simulink model "Parking"  (R2024a)
settings: Solver=VariableStepAuto  StartTime=0.0  StopTime=10.0  RelTol=1e-3
undefined symbols (not defined in the file): Traffic_Info
libraries: CarMaker4SL x56, slpidlib x1
settings Model: Creator=User  LastModifiedBy=User

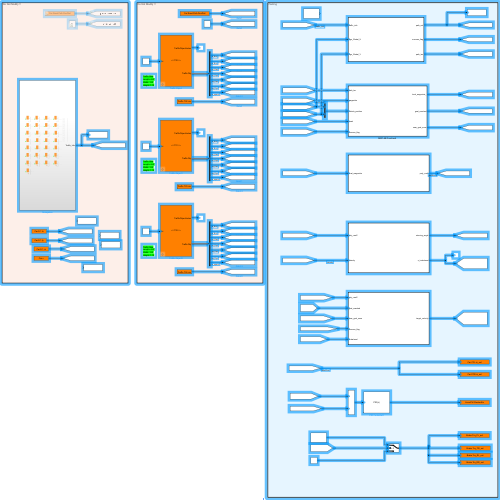
[thumbnail: Simulink's stored preview of the top-level diagram]
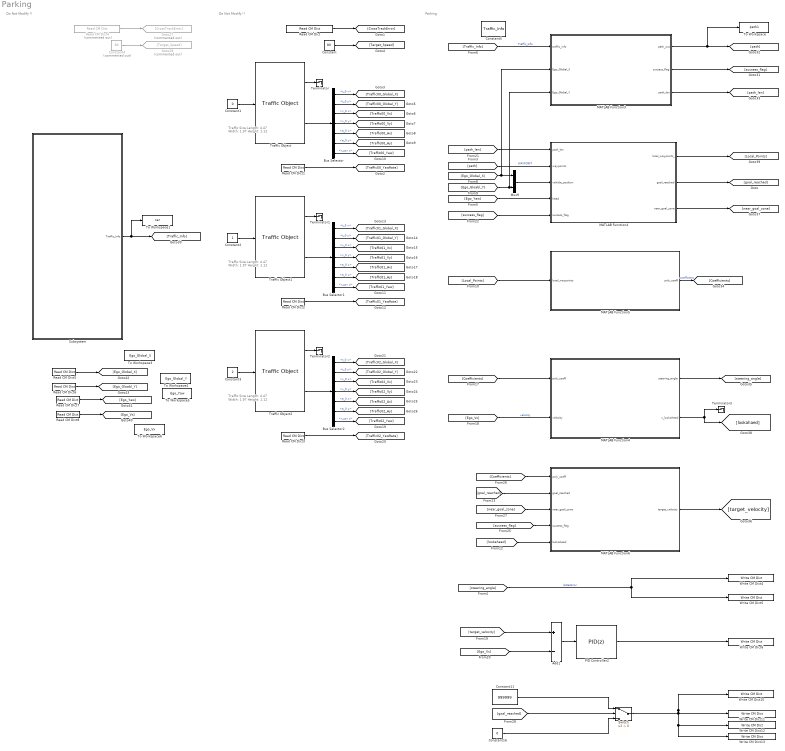
== system Parking ==
  note: Do Not Modify !!
  note: Traffic Size
      | Length: 4.47
      | Width: 1.97
      | Height: 1.12
  note: Traffic Size
      | Length: 4.47
      | Width: 1.97
      | Height: 1.12
  note: Traffic Size
      | Length: 4.47
      | Width: 1.97
      | Height: 1.12
  note: Do Not Modify !!
  note: Parking
  Add1 : Sum  Inputs=+-
  Bus Selector : BusSelector  OutputSignals=t_0 x,t_0 y,v_0 x,v_0 y,a_0 x,a_0 y,r_zyx z
  Bus Selector1 : BusSelector  OutputSignals=t_0 x,t_0 y,v_0 x,v_0 y,a_0 x,a_0 y,r_zyx z
  Bus Selector2 : BusSelector  OutputSignals=t_0 x,t_0 y,v_0 x,v_0 y,a_0 x,a_0 y,r_zyx z
  Constant : Constant  Value=80
  Constant1 : Constant  Value=0
  Constant11 : Constant  Value=999999
  Constant16 : Constant  Value=0
  Constant2 : Constant
  Constant3 : Constant  Value=2
  Constant4 : Constant  Commented=on  Value=80
  Constant5 : Constant  Value=Traffic_Info
  Goto27 : Goto  Commented=on  GotoTag=CrossTrackError
  Goto29 : Goto  Commented=on  GotoTag=Target_Speed
  MATLAB Function3 : MATLAB Function  TreatAsAtomicUnit=on
  MATLAB Function4 : MATLAB Function  TreatAsAtomicUnit=on
  "MATLAB Function4 " : MATLAB Function  TreatAsAtomicUnit=on
  MATLAB Function5 : MATLAB Function  TreatAsAtomicUnit=on
  MATLAB Function6 : MATLAB Function  TreatAsAtomicUnit=on
  Mux9 : Mux  Inputs=2
  PID Controller2 : slpidlib/PID Controller  Controller=PID  Form=Parallel  TimeDomain=Discrete-time  UseExternalTs=off  SampleTime=-1  IntegratorMethod=Forward Euler  FilterMethod=Forward Euler  ControllerParametersSource=internal  P=3  I=0.00  UseKiTs=off  D=0.1  UseExternalDerivativeSource=off  N=100  UseFilter=off  TunerSelectOption=Transfer Function Based (PID Tuner App)  InitialConditionSource=internal  InitialConditionForIntegrator=0  InitialConditionForFilter=0  DifferentiatorICPrevScaledInput=0  ExternalReset=none  TrackingMode=off  Kt=1  LimitOutput=off  SatLimitsSource=internal  UpperSaturationLimit=inf  LowerSaturationLimit=-inf  LinearizeAsGain=on  AntiWindupMode=none  Kb=1  LimitIntegrator=off  UpperIntegratorSaturationLimit=inf  LowerIntegratorSaturationLimit=-inf  POutMin=[]  POutMax=[]  IOutMin=[]  IOutMax=[]  DOutMin=[]  DOutMax=[]  NOutMin=[]  NOutMax=[]  SumOutMin=[]  SumOutMax=[]  SaturationOutMin=[]  SaturationOutMax=[]  PParamMin=[]  PParamMax=[]  IParamMin=[]  IParamMax=[]  DParamMin=[]  DParamMax=[]  NParamMin=[]  NParamMax=[]  KbParamMin=[]  KbParamMax=[]  KtParamMin=[]  KtParamMax=[]  KbOutMin=[]  KbOutMax=[]  KtOutMin=[]  KtOutMax=[]  IntegratorOutMin=[]  IntegratorOutMax=[]  FilterOutMin=[]  FilterOutMax=[]  SumI1OutMin=[]  SumI1OutMax=[]  SumI2OutMin=[]  SumI2OutMax=[]  SumI3OutMin=[]  SumI3OutMax=[]  SumI4OutMin=[]  SumI4OutMax=[]  SumDOutMin=[]  SumDOutMax=[]  DifferentiatorOutMin=[]  DifferentiatorOutMax=[]  FilterDiffOutCoefMin=[]  FilterDiffOutCoefMax=[]  ReciprocalOutMin=[]  ReciprocalOutMax=[]  SumDenOutMin=[]  SumDenOutMax=[]  SumNumOutMin=[]  SumNumOutMax=[]  DivideOutMin=[]  DivideOutMax=[]  UdiffTsProdOutMin=[]  UdiffTsProdOutMax=[]  NTsProdOutMin=[]  NTsProdOutMax=[]  UintegralTsProdOutMin=[]  UintegralTsProdOutMax=[]  UngainTsProdOutMin=[]  UngainTsProdOutMax=[]  ClampingZeroOutDataTypeStr=Inherit: Inherit via back propagation  ClampingZeroOutMin=[]  ClampingZeroOutMax=[]  FilterDenConstantOutDataTypeStr=Inherit: Inherit via back propagation  FilterDenConstantOutMin=[]  FilterDenConstantOutMax=[]  PCopyOutDataTypeStr=Inherit: Inherit via back propagation  PCopyOutMin=[]  PCopyOutMax=[]  NCopyOutDataTypeStr=Inherit: Inherit via back propagation  NCopyOutMin=[]  NCopyOutMax=[]  IntegratorContinuousStateAttributes=''  IntegratorStateMustResolveToSignalObject=off  IntegratorRTWStateStorageClass=Auto  FilterContinuousStateAttributes=''  FilterStateMustResolveToSignalObject=off  FilterRTWStateStorageClass=Auto  ParallelPVariant=InternalParameters  IdealPVariant=Disabled  IVariant=InternalParameters  DVariant=InternalParameters  IntegratorVariant=Discrete  SatVariant=Disabled  AWVariant=Passthrough  PCopyVariant=Disabled  TRVariant=Disabled  FdbkBlocksVariant=Forward  IdealPFdbkVariant=Disabled  SatFdbkVariant=Disabled  DerivativeFilterVariant=Differentiator  NVariant=Passthrough  NCopyVariant=Disabled_SignalSpec  FilterICVariant=InternalICsDifferentiator  IntegratorICVariant=InternalICs  ExternalResetVariant=Disabled  TRSumVariant=Passthrough  SumFdbkVariant=Disabled  SumVariant=Sum_PID  TsampFilterVariant=InternalTs  TsampNgainVariant=Passthrough  TsampIntegralVariant=Disabled_SignalSpec  ExternalSaturationOutDataTypeStr=Inherit: Same as second input  DerivativeSourceVariant=ErrorSignal
  Read CM Dict : CarMaker4SL/Read CM Dict  xname=Car.Road.Path.DevDist  xsync=off  xstime=Inherited
  Read CM Dict1 : CarMaker4SL/Read CM Dict  xname=Traffic.T22.rzv  xsync=off  xstime=Inherited
  Read CM Dict2 : CarMaker4SL/Read CM Dict  xname=Traffic.T23.rzv  xsync=off  xstime=Inherited
  Read CM Dict3 : CarMaker4SL/Read CM Dict  xname=Traffic.T24.rzv  xsync=off  xstime=Inherited
  Read CM Dict4 : CarMaker4SL/Read CM Dict  Commented=on  xname=Car.Road.Path.DevDist  xsync=off  xstime=Inherited
  Read CM Dict5 : CarMaker4SL/Read CM Dict  xname=Car.Fr1.tx  xsync=off  xstime=Inherited
  Read CM Dict6 : CarMaker4SL/Read CM Dict  xname=Car.Fr1.ty  xsync=off  xstime=Inherited
  Read CM Dict7 : CarMaker4SL/Read CM Dict  xname=Car.Fr1.rz  xsync=off  xstime=Inherited
  Read CM Dict8 : CarMaker4SL/Read CM Dict  xname=Car.v  xsync=off  xstime=Inherited
  Subsystem : Subsystem
  Switch : Switch  Criteria=u2 > Threshold  SaturateOnIntegerOverflow=off  InputSameDT=off
  Terminator{,1..3} (4 alike) : Terminator
  To Workspace : ToWorkspace  VariableName=path1  SaveFormat=Structure With Time  SampleTime=-1
  To Workspace1 : ToWorkspace  VariableName=car  SaveFormat=Timeseries  SampleTime=-1
  To Workspace3 : ToWorkspace  VariableName=Ego_Global_X  SaveFormat=Structure With Time  SampleTime=-1
  To Workspace4 : ToWorkspace  VariableName=Ego_Global_Y  SaveFormat=Structure With Time  SampleTime=-1
  To Workspace5 : ToWorkspace  VariableName=Ego_Yaw  SaveFormat=Structure With Time  SampleTime=-1
  To Workspace6 : ToWorkspace  VariableName=Ego_Vx  SaveFormat=Structure With Time  SampleTime=-1
  Traffic Object : CarMaker4SL/Traffic Object  xname=T00  ximode=Traffic Id  xstime=Inherited
      settings: SourceProductName=CarMaker4SL
  Traffic Object1 : CarMaker4SL/Traffic Object  xname=T01  ximode=Traffic Id  xstime=Inherited
      settings: SourceProductName=CarMaker4SL
  Traffic Object2 : CarMaker4SL/Traffic Object  xname=T02  ximode=Traffic Id  xstime=Inherited
      settings: SourceProductName=CarMaker4SL
  Write CM Dict10 : CarMaker4SL/Write CM Dict  xname=Brake.Trq_FL_ext  xsync=off
  Write CM Dict11 : CarMaker4SL/Write CM Dict  xname=Brake.Trq_FR_ext  xsync=off
  Write CM Dict12 : CarMaker4SL/Write CM Dict  xname=Brake.Trq_RL_ext  xsync=off
  Write CM Dict13 : CarMaker4SL/Write CM Dict  xname=Brake.Trq_RR_ext  xsync=off
  Write CM Dict4 : CarMaker4SL/Write CM Dict  xname=Car.CFL.rz_ext  xsync=off
  Write CM Dict5 : CarMaker4SL/Write CM Dict  xname=Car.CFR.rz_ext  xsync=off
  Write CM Dict6 : CarMaker4SL/Write CM Dict  xname=AccelCtrl.DesiredAx  xsync=off
  wires:
  [steering_angle] -> Write CM Dict5/1, Write CM Dict4/1  "latterError"
  [Traffic_Info] -> MATLAB Function3/1(traffic_info)  "Traffic_Info"
  [Ego_Yaw] -> "MATLAB Function4 "/4(head)
  [Coefficients] -> MATLAB Function4/1(poly_coeff)
  Traffic Object2/1 -> Terminator2/1
  Read CM Dict5/1 -> [Ego_Global_X]
  Constant11/1 -> Switch/1
  [success_flag] -> "MATLAB Function4 "/5(success_flag)
  Bus Selector1/1 -> [Traffic01_Global_X]  "<t_0 x>"
  [goal_reached] -> MATLAB Function6/2(goal_reached)
  [success_flag] -> MATLAB Function6/4(success_flag)
  Constant16/1 -> Switch/3
  Read CM Dict8/1 -> [Ego_Vx]
  Read CM Dict3/1 -> [Traffic02_YawRate]
  MATLAB Function3/3(path_len) -> [path_len]
  "MATLAB Function4 "/1(local_waypoints_) -> [Local_Points]
  MATLAB Function5/1(poly_coeff) -> [Coefficients]  "coefficient"
  Bus Selector2/3 -> [Traffic02_Vx]  "<v_0 x>"
  Subsystem/1(Traffic_Info) -> To Workspace1/1, [Traffic_Info]
  [Coefficients] -> MATLAB Function6/1(poly_coeff)
  Bus Selector/6 -> [Traffic00_Ay]  "<a_0 y>"
  Constant4/1 -> Goto29/1
  Bus Selector2/6 -> [Traffic02_Ay]  "<a_0 y>"
  [path_len] -> "MATLAB Function4 "/1(path_len)
  Add1/1 -> PID Controller2/1
  Traffic Object/1 -> Terminator/1
  MATLAB Function3/2(success_flag) -> [success_flag]
  Bus Selector1/5 -> [Traffic01_Ax]  "<a_0 x>"
  [path] -> "MATLAB Function4 "/2(waypoints)  "WAYPOINT"
  Read CM Dict7/1 -> [Ego_Yaw]
  MATLAB Function4/2(x_lookahead) -> Terminator3/1, [lookahaed]
  Bus Selector1/3 -> [Traffic01_Vx]  "<v_0 x>"
  MATLAB Function6/1(target_velocity) -> [target_velocity]
  [target_velocity] -> Add1/1
  Mux9/1 -> "MATLAB Function4 "/3(vehicle_position)
  "MATLAB Function4 "/2(goal_reached) -> [goal_reached]
  [near_goal_zone] -> MATLAB Function6/3(near_goal_zone)
  Constant3/1 -> Traffic Object2/1
  Bus Selector2/2 -> [Traffic02_Global_Y]  "<t_0 y>"
  [Ego_Global_X] -> MATLAB Function3/2(Ego_Global_X), Mux9/1
  "MATLAB Function4 "/3(near_goal_zone) -> [near_goal_zone]
  Read CM Dict6/1 -> [Ego_Gloabl_Y]
  Read CM Dict2/1 -> [Traffic01_YawRate]
  [Ego_Vx] -> Add1/2
  Bus Selector/7 -> [Traffic00_Yaw]  "<r_zyx z>"
  Bus Selector2/5 -> [Traffic02_Ax]  "<a_0 x>"
  [goal_reached] -> Switch/2
  Traffic Object1/2 -> Bus Selector1/1
  Traffic Object1/1 -> Terminator1/1
  Bus Selector/2 -> [Traffic00_Global_Y]  "<t_0 y>"
  [lookahaed] -> MATLAB Function6/5(lookahead)
  Bus Selector/1 -> [Traffic00_Global_X]  "<t_0 x>"
  [Local_Points] -> MATLAB Function5/1(local_waypoints)
  Bus Selector1/4 -> [Traffic01_Vy]  "<v_0 y>"
  MATLAB Function4/1(steering_angle) -> [steering_angle]
  Traffic Object2/2 -> Bus Selector2/1
  Read CM Dict4/1 -> Goto27/1
  Constant2/1 -> Traffic Object1/1
  Bus Selector1/2 -> [Traffic01_Global_Y]  "<t_0 y>"
  Bus Selector2/1 -> [Traffic02_Global_X]  "<t_0 x>"
  Bus Selector1/6 -> [Traffic01_Ay]  "<a_0 y>"
  Switch/1 -> Write CM Dict13/1, Write CM Dict12/1, Write CM Dict10/1, Write CM Dict11/1
  Bus Selector/5 -> [Traffic00_Ax]  "<a_0 x>"
  MATLAB Function3/1(path_out) -> To Workspace/1, [path]
  Bus Selector2/7 -> [Traffic02_Yaw]  "<r_zyx z>"
  [Ego_Vx] -> MATLAB Function4/2(velocity)  "velocity"
  Bus Selector2/4 -> [Traffic02_Vy]  "<v_0 y>"
  Bus Selector1/7 -> [Traffic01_Yaw]  "<r_zyx z>"
  Bus Selector/4 -> [Traffic00_Vy]  "<v_0 y>"
  Read CM Dict/1 -> [CrossTrackError]
  Read CM Dict1/1 -> [Traffic00_YawRate]
  Traffic Object/2 -> Bus Selector/1
  Bus Selector/3 -> [Traffic00_Vx]  "<v_0 x>"
  PID Controller2/1 -> Write CM Dict6/1
  Constant/1 -> [Target_Speed]
  [Ego_Gloabl_Y] -> MATLAB Function3/3(Ego_Global_Y), Mux9/2
  Constant1/1 -> Traffic Object/1

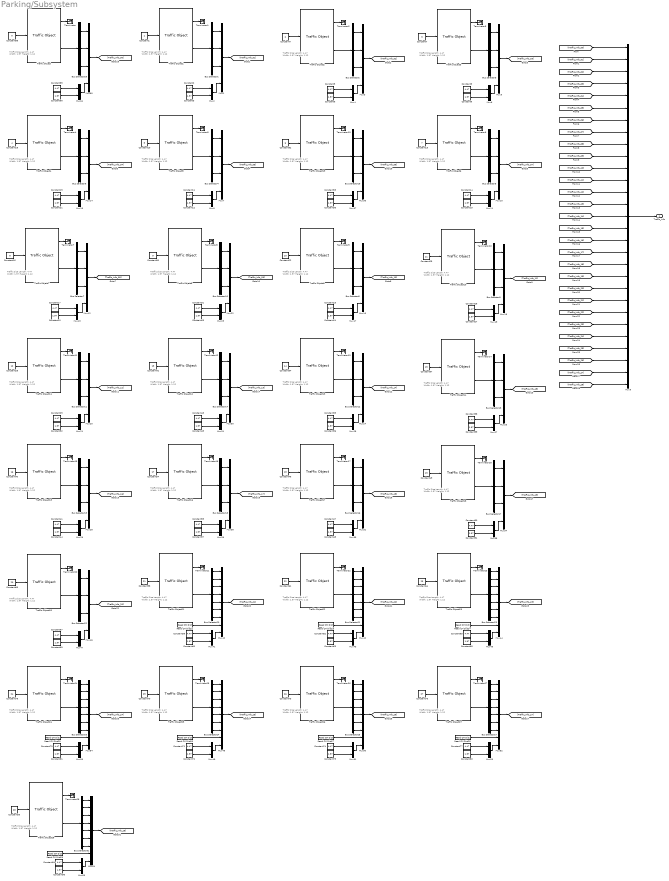
== system Parking/Subsystem ==
  note: Traffic Size
      | Length: 4.47
      | Width: 1.97
      | Height: 1.12
  note: Traffic Size
      | Length: 4.47
      | Width: 1.97
      | Height: 1.12
  note: Traffic Size
      | Length: 4.47
      | Width: 1.97
      | Height: 1.12
  note: Traffic Size
      | Length: 4.47
      | Width: 1.97
      | Height: 1.12
  note: Traffic Size
      | Length: 4.47
      | Width: 1.97
      | Height: 1.12
  note: Traffic Size
      | Length: 4.47
      | Width: 1.97
      | Height: 1.12
  note: Traffic Size
      | Length: 4.47
      | Width: 1.97
      | Height: 1.12
  note: Traffic Size
      | Length: 4.47
      | Width: 1.97
      | Height: 1.12
  note: Traffic Size
      | Length: 4.47
      | Width: 1.97
      | Height: 1.12
  note: Traffic Size
      | Length: 4.47
      | Width: 1.97
      | Height: 1.12
  note: Traffic Size
      | Length: 4.47
      | Width: 1.97
      | Height: 1.12
  note: Traffic Size
      | Length: 4.47
      | Width: 1.97
      | Height: 1.12
  note: Traffic Size
      | Length: 4.47
      | Width: 1.97
      | Height: 1.12
  note: Traffic Size
      | Length: 4.47
      | Width: 1.97
      | Height: 1.12
  note: Traffic Size
      | Length: 4.47
      | Width: 1.97
      | Height: 1.12
  note: Traffic Size
      | Length: 4.47
      | Width: 1.97
      | Height: 1.12
  note: Traffic Size
      | Length: 4.47
      | Width: 1.97
      | Height: 1.12
  note: Traffic Size
      | Length: 4.47
      | Width: 1.97
      | Height: 1.12
  note: Traffic Size
      | Length: 4.47
      | Width: 1.97
      | Height: 1.12
  note: Traffic Size
      | Length: 4.47
      | Width: 1.97
      | Height: 1.12
  note: Traffic Size
      | Length: 4.47
      | Width: 1.97
      | Height: 1.12
  note: Traffic Size
      | Length: 4.47
      | Width: 1.97
      | Height: 1.12
  note: Traffic Size
      | Length: 4.47
      | Width: 1.97
      | Height: 1.12
  note: Traffic Size
      | Length: 4.47
      | Width: 1.97
      | Height: 1.12
  note: Traffic Size
      | Length: 4.47
      | Width: 1.97
      | Height: 1.12
  note: Traffic Size
      | Length: 4.47
      | Width: 1.97
      | Height: 1.12
  note: Traffic Size
      | Length: 4.47
      | Width: 1.97
      | Height: 1.12
  note: Traffic Size
      | Length: 4.47
      | Width: 1.97
      | Height: 1.12
  note: Traffic Size
      | Length: 4.47
      | Width: 1.97
      | Height: 1.12
  Bus Selector{1..19,22,29} (21 alike) : BusSelector  OutputSignals=t_0 x,t_0 y,r_zyx z
  Bus Selector{20..21,23..27,31} (8 alike) : BusSelector  OutputSignals=t_0 x,t_0 y,v_0 x,v_0 y,a_0 x,a_0 y,r_zyx z
  Constant1 : Constant
  Constant10 : Constant  Value=5
  Constant{2,5,8,11,14,17,19,23,26,29,31,35,38,41,43,47,50,53,55,59,62,65,67,71,74,77,79,89,94} (29 alike) : Constant  Value=4.47
  Constant{3,6,9,12,15,20..21,24,27,32..33,36,39,44..45,48,51,56..57,60,63,68..69,72,75,80..81,90,96} (29 alike) : Constant  Value=1.97
  Constant13 : Constant  Value=7
  Constant16 : Constant  Value=8
  Constant18 : Constant  Value=4
  Constant22 : Constant  Value=10
  Constant25 : Constant  Value=11
  Constant28 : Constant  Value=12
  Constant30 : Constant  Value=9
  Constant34 : Constant  Value=14
  Constant37 : Constant  Value=15
  Constant4 : Constant  Value=2
  Constant40 : Constant  Value=16
  Constant42 : Constant  Value=13
  Constant46 : Constant  Value=18
  Constant49 : Constant  Value=19
  Constant52 : Constant  Value=6
  Constant54 : Constant  Value=17
  Constant58 : Constant  Value=21
  Constant61 : Constant  Value=22
  Constant64 : Constant  Value=23
  Constant66 : Constant  Value=20
  Constant7 : Constant  Value=3
  Constant70 : Constant  Value=25
  Constant73 : Constant  Value=26
  Constant76 : Constant  Value=27
  Constant78 : Constant  Value=24
  Constant88 : Constant  Value=0
  Constant93 : Constant  Value=28
  Mux{1,3,5,7,10,12,14,16,18,20,22,24,26,28,30,32,34,36,38,46,60} (21 alike) : Mux
  Mux{2,4,6,8,11,13,15,17,19,21,23,25,27,29,31,33,35,37,39,41,43,45,47,49,51,53,55,61,65} (29 alike) : Mux  Inputs=2
  Mux{40,42,44,48,50,52,54,64} (8 alike) : Mux  Inputs=9
  Mux9 : Mux  Inputs=29
  Read CM Dict22 : CarMaker4SL/Read CM Dict  xname=Traffic.T21.rzv  xsync=off  xstime=Inherited
  Read CM Dict23 : CarMaker4SL/Read CM Dict  xname=Traffic.T22.rzv  xsync=off  xstime=Inherited
  Read CM Dict24 : CarMaker4SL/Read CM Dict  xname=Traffic.T23.rzv  xsync=off  xstime=Inherited
  Read CM Dict25 : CarMaker4SL/Read CM Dict  xname=Traffic.T24.rzv  xsync=off  xstime=Inherited
  Read CM Dict26 : CarMaker4SL/Read CM Dict  xname=Traffic.T25.rzv  xsync=off  xstime=Inherited
  Read CM Dict27 : CarMaker4SL/Read CM Dict  xname=Traffic.T26.rzv  xsync=off  xstime=Inherited
  Read CM Dict28 : CarMaker4SL/Read CM Dict  xname=Traffic.T27.rzv  xsync=off  xstime=Inherited
  Read CM Dict29 : CarMaker4SL/Read CM Dict  xname=Traffic.T28.rzv  xsync=off  xstime=Inherited
  Terminator{,1..28} (29 alike) : Terminator
  Traffic Object : CarMaker4SL/Traffic Object  xname=T00  ximode=Traffic Id  xstime=Inherited
      settings: SourceProductName=CarMaker4SL
  Traffic Object1 : CarMaker4SL/Traffic Object  xname=T01  ximode=Traffic Id  xstime=Inherited
      settings: SourceProductName=CarMaker4SL
  Traffic Object10 : CarMaker4SL/Traffic Object  xname=T11  ximode=Traffic Id  xstime=Inherited
      settings: SourceProductName=CarMaker4SL
  Traffic Object11 : CarMaker4SL/Traffic Object  xname=T12  ximode=Traffic Id  xstime=Inherited
      settings: SourceProductName=CarMaker4SL
  Traffic Object12 : CarMaker4SL/Traffic Object  xname=T13  ximode=Traffic Id  xstime=Inherited
      settings: SourceProductName=CarMaker4SL
  Traffic Object13 : CarMaker4SL/Traffic Object  xname=T14  ximode=Traffic Id  xstime=Inherited
      settings: SourceProductName=CarMaker4SL
  Traffic Object14 : CarMaker4SL/Traffic Object  xname=T15  ximode=Traffic Id  xstime=Inherited
      settings: SourceProductName=CarMaker4SL
  Traffic Object15 : CarMaker4SL/Traffic Object  xname=T16  ximode=Traffic Id  xstime=Inherited
      settings: SourceProductName=CarMaker4SL
  Traffic Object16 : CarMaker4SL/Traffic Object  xname=T17  ximode=Traffic Id  xstime=Inherited
      settings: SourceProductName=CarMaker4SL
  Traffic Object17 : CarMaker4SL/Traffic Object  xname=T18  ximode=Traffic Id  xstime=Inherited
      settings: SourceProductName=CarMaker4SL
  Traffic Object18 : CarMaker4SL/Traffic Object  xname=T19  ximode=Traffic Id  xstime=Inherited
      settings: SourceProductName=CarMaker4SL
  Traffic Object19 : CarMaker4SL/Traffic Object  xname=T06  ximode=Traffic Id  xstime=Inherited
      settings: SourceProductName=CarMaker4SL
  Traffic Object2 : CarMaker4SL/Traffic Object  xname=T02  ximode=Traffic Id  xstime=Inherited
      settings: SourceProductName=CarMaker4SL
  Traffic Object20 : CarMaker4SL/Traffic Object  xname=T20  ximode=Traffic Id  xstime=Inherited
      settings: SourceProductName=CarMaker4SL
  Traffic Object21 : CarMaker4SL/Traffic Object  xname=T21  ximode=Traffic Id  xstime=Inherited
      settings: SourceProductName=CarMaker4SL
  Traffic Object22 : CarMaker4SL/Traffic Object  xname=T22  ximode=Traffic Id  xstime=Inherited
      settings: SourceProductName=CarMaker4SL
  Traffic Object23 : CarMaker4SL/Traffic Object  xname=T23  ximode=Traffic Id  xstime=Inherited
      settings: SourceProductName=CarMaker4SL
  Traffic Object24 : CarMaker4SL/Traffic Object  xname=T24  ximode=Traffic Id  xstime=Inherited
      settings: SourceProductName=CarMaker4SL
  Traffic Object25 : CarMaker4SL/Traffic Object  xname=T25  ximode=Traffic Id  xstime=Inherited
      settings: SourceProductName=CarMaker4SL
  Traffic Object26 : CarMaker4SL/Traffic Object  xname=T26  ximode=Traffic Id  xstime=Inherited
      settings: SourceProductName=CarMaker4SL
  Traffic Object27 : CarMaker4SL/Traffic Object  xname=T27  ximode=Traffic Id  xstime=Inherited
      settings: SourceProductName=CarMaker4SL
  Traffic Object28 : CarMaker4SL/Traffic Object  xname=T28  ximode=Traffic Id  xstime=Inherited
      settings: SourceProductName=CarMaker4SL
  Traffic Object3 : CarMaker4SL/Traffic Object  xname=T03  ximode=Traffic Id  xstime=Inherited
      settings: SourceProductName=CarMaker4SL
  Traffic Object4 : CarMaker4SL/Traffic Object  xname=T04  ximode=Traffic Id  xstime=Inherited
      settings: SourceProductName=CarMaker4SL
  Traffic Object5 : CarMaker4SL/Traffic Object  xname=T05  ximode=Traffic Id  xstime=Inherited
      settings: SourceProductName=CarMaker4SL
  Traffic Object6 : CarMaker4SL/Traffic Object  xname=T07  ximode=Traffic Id  xstime=Inherited
      settings: SourceProductName=CarMaker4SL
  Traffic Object7 : CarMaker4SL/Traffic Object  xname=T08  ximode=Traffic Id  xstime=Inherited
      settings: SourceProductName=CarMaker4SL
  Traffic Object8 : CarMaker4SL/Traffic Object  xname=T09  ximode=Traffic Id  xstime=Inherited
      settings: SourceProductName=CarMaker4SL
  Traffic Object9 : CarMaker4SL/Traffic Object  xname=T10  ximode=Traffic Id  xstime=Inherited
      settings: SourceProductName=CarMaker4SL
  Traffic_Info : Outport
  wires:
  Constant94/1 -> Mux65/1
  [Traffic_Info_28] -> Mux9/29
  Mux22/1 -> [Traffic_Info_09]
  Constant16/1 -> Traffic Object7/1
  Mux11/1 -> Mux10/4
  Bus Selector7/1 -> Mux12/1  "<t_0 x>"
  Bus Selector4/3 -> Mux7/3  "<r_zyx z>"
  Constant3/1 -> Mux2/2
  Mux12/1 -> [Traffic_Info_08]
  Traffic Object5/2 -> Bus Selector4/1
  Constant1/1 -> Traffic Object1/1
  Traffic Object7/2 -> Bus Selector7/1
  Traffic Object4/2 -> Bus Selector6/1
  Constant12/1 -> Mux8/2
  Constant19/1 -> Mux15/1
  Constant11/1 -> Mux8/1
  Bus Selector6/2 -> Mux14/2  "<t_0 y>"
  Bus Selector23/3 -> Mux44/3  "<v_0 x>"
  Traffic Object8/1 -> Terminator8/1
  Mux15/1 -> Mux14/4
  Mux13/1 -> Mux12/4
  Traffic Object26/2 -> Bus Selector25/1
  Traffic Object4/1 -> Terminator4/1
  Bus Selector23/4 -> Mux44/4  "<v_0 y>"
  Traffic Object23/2 -> Bus Selector23/1
  Bus Selector20/5 -> Mux40/5  "<a_0 x>"
  Constant71/1 -> Mux49/1
  Constant9/1 -> Mux6/2
  Constant6/1 -> Mux4/2
  Traffic Object27/1 -> Terminator27/1
  Traffic Object2/2 -> Bus Selector2/1
  Mux8/1 -> Mux7/4
  Mux5/1 -> [Traffic_Info_03]
  Constant89/1 -> Mux61/1
  [Traffic_Info_06] -> Mux9/7
  Constant7/1 -> Traffic Object3/1
  Bus Selector2/2 -> Mux3/2  "<t_0 y>"
  Bus Selector1/2 -> Mux1/2  "<t_0 y>"
  Read CM Dict25/1 -> Mux54/8
  Bus Selector24/1 -> Mux48/1  "<t_0 x>"
  Mux65/1 -> Mux64/9
  Bus Selector23/5 -> Mux44/5  "<a_0 x>"
  Bus Selector2/1 -> Mux3/1  "<t_0 x>"
  Constant96/1 -> Mux65/2
  Bus Selector24/7 -> Mux48/7  "<r_zyx z>"
  Bus Selector2/3 -> Mux3/3  "<r_zyx z>"
  Bus Selector31/1 -> Mux64/1  "<t_0 x>"
  Constant34/1 -> Traffic Object13/1
  Bus Selector20/4 -> Mux40/4  "<v_0 y>"
  Mux31/1 -> Mux30/4
  Traffic Object12/2 -> Bus Selector14/1
  Bus Selector10/1 -> Mux22/1  "<t_0 x>"
  Bus Selector27/4 -> Mux52/4  "<v_0 y>"
  Traffic Object25/1 -> Terminator25/1
  Mux21/1 -> Mux20/4
  Bus Selector23/7 -> Mux44/7  "<r_zyx z>"
  Mux14/1 -> [Traffic_Info_04]
  Constant42/1 -> Traffic Object12/1
  Constant43/1 -> Mux31/1
  Constant36/1 -> Mux25/2
  [Traffic_Info_02] -> Mux9/3
  Bus Selector24/4 -> Mux48/4  "<v_0 y>"
  Mux25/1 -> Mux24/4
  [Traffic_Info_05] -> Mux9/6
  Traffic Object9/2 -> Bus Selector8/1
  Constant26/1 -> Mux19/1
  Bus Selector9/2 -> Mux18/2  "<t_0 y>"
  Read CM Dict27/1 -> Mux50/8
  Traffic Object1/2 -> Bus Selector1/1
  Mux4/1 -> Mux3/4
  Constant70/1 -> Traffic Object25/1
  Mux50/1 -> [Traffic_Info_26]
  Constant72/1 -> Mux49/2
  Bus Selector11/2 -> Mux20/2  "<t_0 y>"
  Traffic Object10/1 -> Terminator10/1
  Constant31/1 -> Mux23/1
  Constant60/1 -> Mux41/2
  Traffic Object8/2 -> Bus Selector10/1
  Bus Selector4/1 -> Mux7/1  "<t_0 x>"
  Mux20/1 -> [Traffic_Info_12]
  Bus Selector23/1 -> Mux44/1  "<t_0 x>"
  Mux23/1 -> Mux22/4
  Constant2/1 -> Mux2/1
  Bus Selector8/3 -> Mux16/3  "<r_zyx z>"
  Mux40/1 -> [Traffic_Info_21]
  Bus Selector20/6 -> Mux40/6  "<a_0 y>"
  Constant22/1 -> Traffic Object9/1
  Constant15/1 -> Mux11/2
  Bus Selector1/3 -> Mux1/3  "<r_zyx z>"
  [Traffic_Info_00] -> Mux9/1
  Mux17/1 -> Mux16/4
  Bus Selector18/3 -> Mux38/3  "<r_zyx z>"
  Mux10/1 -> [Traffic_Info_07]
  Bus Selector27/7 -> Mux52/7  "<r_zyx z>"
  [Traffic_Info_04] -> Mux9/5
  Mux28/1 -> [Traffic_Info_16]
  Traffic Object11/2 -> Bus Selector11/1
  Constant8/1 -> Mux6/1
  Constant45/1 -> Mux31/2
  Traffic Object9/1 -> Terminator9/1
  Constant23/1 -> Mux17/1
  Bus Selector8/2 -> Mux16/2  "<t_0 y>"
  Mux29/1 -> Mux28/4
  Bus Selector13/2 -> Mux26/2  "<t_0 y>"
  Bus Selector31/4 -> Mux64/4  "<v_0 y>"
  Bus Selector3/3 -> Mux5/3  "<r_zyx z>"
  [Traffic_Info_22] -> Mux9/23
  Traffic Object13/2 -> Bus Selector12/1
  Bus Selector10/3 -> Mux22/3  "<r_zyx z>"
  [Traffic_Info_21] -> Mux9/22
  Bus Selector24/5 -> Mux48/5  "<a_0 x>"
  Mux64/1 -> [Traffic_Info_28]
  Bus Selector15/2 -> Mux28/2  "<t_0 y>"
  [Traffic_Info_16] -> Mux9/17
  Bus Selector29/1 -> Mux60/1  "<t_0 x>"
  Traffic Object14/1 -> Terminator14/1
  Constant44/1 -> Mux29/2
  Constant38/1 -> Mux27/1
  Bus Selector21/3 -> Mux42/3  "<v_0 x>"
  Mux43/1 -> Mux42/9
  Traffic Object13/1 -> Terminator13/1
  Constant4/1 -> Traffic Object2/1
  Constant40/1 -> Traffic Object15/1
  Constant39/1 -> Mux27/2
  Constant25/1 -> Traffic Object10/1
  Mux53/1 -> Mux52/9
  Mux16/1 -> [Traffic_Info_10]
  Read CM Dict24/1 -> Mux44/8
  Constant13/1 -> Traffic Object6/1
  Bus Selector26/7 -> Mux54/7  "<r_zyx z>"
  Constant75/1 -> Mux51/2
  Mux49/1 -> Mux48/9
  Traffic Object21/2 -> Bus Selector20/1
  Constant27/1 -> Mux19/2
  Traffic Object26/1 -> Terminator26/1
  Mux1/1 -> [Traffic_Info_01]
  Bus Selector26/5 -> Mux54/5  "<a_0 x>"
  Bus Selector27/5 -> Mux52/5  "<a_0 x>"
  Traffic Object2/1 -> Terminator2/1
  Constant65/1 -> Mux45/1
  Constant33/1 -> Mux23/2
  Read CM Dict22/1 -> Mux40/8
  Constant62/1 -> Mux43/1
  Bus Selector26/1 -> Mux54/1  "<t_0 x>"
  Read CM Dict23/1 -> Mux42/8
  Bus Selector21/7 -> Mux42/7  "<r_zyx z>"
  Traffic Object3/2 -> Bus Selector3/1
  Bus Selector20/1 -> Mux40/1  "<t_0 x>"
  Mux18/1 -> [Traffic_Info_11]
  [Traffic_Info_13] -> Mux9/14
  Bus Selector20/3 -> Mux40/3  "<v_0 x>"
  Traffic Object21/1 -> Terminator21/1
  Bus Selector26/3 -> Mux54/3  "<v_0 x>"
  Constant59/1 -> Mux41/1
  Bus Selector21/4 -> Mux42/4  "<v_0 y>"
  [Traffic_Info_11] -> Mux9/12
  Mux44/1 -> [Traffic_Info_23]
  Bus Selector23/6 -> Mux44/6  "<a_0 y>"
  Mux42/1 -> [Traffic_Info_22]
  Traffic Object22/2 -> Bus Selector21/1
  Bus Selector23/2 -> Mux44/2  "<t_0 y>"
  Mux45/1 -> Mux44/9
  Bus Selector5/1 -> Mux10/1  "<t_0 x>"
  Bus Selector21/5 -> Mux42/5  "<a_0 x>"
  Traffic Object23/1 -> Terminator23/1
  Constant58/1 -> Traffic Object21/1
  Bus Selector29/3 -> Mux60/3  "<r_zyx z>"
  [Traffic_Info_03] -> Mux9/4
  [Traffic_Info_25] -> Mux9/26
  Bus Selector29/2 -> Mux60/2  "<t_0 y>"
  Constant90/1 -> Mux61/2
  Traffic Object/1 -> Terminator/1
  [Traffic_Info_17] -> Mux9/18
  Mux41/1 -> Mux40/9
  [Traffic_Info_18] -> Mux9/19
  Mux60/1 -> [Traffic_Info_00]
  [Traffic_Info_07] -> Mux9/8
  Traffic Object/2 -> Bus Selector29/1
  Bus Selector31/3 -> Mux64/3  "<v_0 x>"
  Constant79/1 -> Mux55/1
  Bus Selector25/4 -> Mux50/4  "<v_0 y>"
  Mux30/1 -> [Traffic_Info_13]
  Bus Selector31/6 -> Mux64/6  "<a_0 y>"
  Constant76/1 -> Traffic Object27/1
  Read CM Dict26/1 -> Mux48/8
  Mux54/1 -> [Traffic_Info_24]
  Bus Selector21/1 -> Mux42/1  "<t_0 x>"
  Constant81/1 -> Mux55/2
  Traffic Object5/1 -> Terminator5/1
  Bus Selector26/2 -> Mux54/2  "<t_0 y>"
  Bus Selector9/3 -> Mux18/3  "<r_zyx z>"
  Traffic Object15/2 -> Bus Selector15/1
  Bus Selector25/7 -> Mux50/7  "<r_zyx z>"
  Bus Selector31/2 -> Mux64/2  "<t_0 y>"
  Bus Selector27/1 -> Mux52/1  "<t_0 x>"
  Mux61/1 -> Mux60/4
  Bus Selector25/1 -> Mux50/1  "<t_0 x>"
  Traffic Object27/2 -> Bus Selector27/1
  Bus Selector25/6 -> Mux50/6  "<a_0 y>"
  Bus Selector26/4 -> Mux54/4  "<v_0 y>"
  Constant20/1 -> Mux13/2
  Mux24/1 -> [Traffic_Info_14]
  Bus Selector25/3 -> Mux50/3  "<v_0 x>"
  Traffic Object7/1 -> Terminator7/1
  Mux39/1 -> Mux38/4
  Bus Selector16/1 -> Mux32/1  "<t_0 x>"
  [Traffic_Info_14] -> Mux9/15
  Constant47/1 -> Mux33/1
  Constant35/1 -> Mux25/1
  Constant74/1 -> Mux51/1
  Bus Selector17/2 -> Mux34/2  "<t_0 y>"
  Bus Selector24/3 -> Mux48/3  "<v_0 x>"
  Traffic Object25/2 -> Bus Selector24/1
  Constant68/1 -> Mux45/2
  Bus Selector25/5 -> Mux50/5  "<a_0 x>"
  Constant5/1 -> Mux4/1
  Traffic Object14/2 -> Bus Selector13/1
  Bus Selector6/3 -> Mux14/3  "<r_zyx z>"
  Bus Selector31/5 -> Mux64/5  "<a_0 x>"
  Constant29/1 -> Mux21/1
  Traffic Object6/2 -> Bus Selector5/1
  Traffic Object18/2 -> Bus Selector17/1
  Bus Selector9/1 -> Mux18/1  "<t_0 x>"
  Mux52/1 -> [Traffic_Info_27]
  Constant61/1 -> Traffic Object22/1
  Mux27/1 -> Mux26/4
  Mux19/1 -> Mux18/4
  Bus Selector21/6 -> Mux42/6  "<a_0 y>"
  Constant54/1 -> Traffic Object16/1
  Bus Selector24/2 -> Mux48/2  "<t_0 y>"
  Traffic Object16/1 -> Terminator16/1
  Bus Selector17/1 -> Mux34/1  "<t_0 x>"
  Traffic Object3/1 -> Terminator3/1
  Mux6/1 -> Mux5/4
  Traffic Object11/1 -> Terminator11/1
  Constant78/1 -> Traffic Object24/1
  Constant57/1 -> Mux39/2
  Constant55/1 -> Mux39/1
  [Traffic_Info_27] -> Mux9/28
  Bus Selector5/3 -> Mux10/3  "<r_zyx z>"
  Traffic Object16/2 -> Bus Selector18/1
  [Traffic_Info_12] -> Mux9/13
  Bus Selector14/1 -> Mux30/1  "<t_0 x>"
  Constant41/1 -> Mux29/1
  Constant93/1 -> Traffic Object28/1
  Bus Selector31/7 -> Mux64/7  "<r_zyx z>"
  Bus Selector17/3 -> Mux34/3  "<r_zyx z>"
  Constant88/1 -> Traffic Object/1
  Mux3/1 -> [Traffic_Info_02]
  Mux9/1 -> Traffic_Info/1
  Constant67/1 -> Mux47/1
  [Traffic_Info_24] -> Mux9/25
  Traffic Object20/1 -> Terminator20/1
  Mux38/1 -> [Traffic_Info_17]
  Traffic Object18/1 -> Terminator18/1
  Constant66/1 -> Traffic Object20/1
  Bus Selector1/1 -> Mux1/1  "<t_0 x>"
  Constant56/1 -> Mux37/2
  Bus Selector22/1 -> Mux46/1  "<t_0 x>"
  Mux34/1 -> [Traffic_Info_19]
  Constant14/1 -> Mux11/1
  Mux46/1 -> [Traffic_Info_20]
  Mux47/1 -> Mux46/4
  Bus Selector22/3 -> Mux46/3  "<r_zyx z>"
  Bus Selector12/1 -> Mux24/1  "<t_0 x>"
  Bus Selector26/6 -> Mux54/6  "<a_0 y>"
  Bus Selector16/3 -> Mux32/3  "<r_zyx z>"
  Bus Selector13/1 -> Mux26/1  "<t_0 x>"
  Traffic Object24/1 -> Terminator24/1
  Traffic Object15/1 -> Terminator15/1
  Traffic Object22/1 -> Terminator22/1
  Constant32/1 -> Mux21/2
  Traffic Object20/2 -> Bus Selector22/1
  Bus Selector21/2 -> Mux42/2  "<t_0 y>"
  Bus Selector7/3 -> Mux12/3  "<r_zyx z>"
  Constant28/1 -> Traffic Object11/1
  Bus Selector14/2 -> Mux30/2  "<t_0 y>"
  Bus Selector22/2 -> Mux46/2  "<t_0 y>"
  Constant48/1 -> Mux33/2
  Bus Selector12/3 -> Mux24/3  "<r_zyx z>"
  Constant49/1 -> Traffic Object18/1
  Mux35/1 -> Mux34/4
  Mux33/1 -> Mux32/4
  Bus Selector20/2 -> Mux40/2  "<t_0 y>"
  Constant69/1 -> Mux47/2
  Bus Selector11/1 -> Mux20/1  "<t_0 x>"
  Traffic Object10/2 -> Bus Selector9/1
  Bus Selector19/3 -> Mux36/3  "<r_zyx z>"
  Bus Selector27/6 -> Mux52/6  "<a_0 y>"
  Constant77/1 -> Mux53/1
  Read CM Dict29/1 -> Mux64/8
  Bus Selector12/2 -> Mux24/2  "<t_0 y>"
  Bus Selector5/2 -> Mux10/2  "<t_0 y>"
  Mux26/1 -> [Traffic_Info_15]
  Read CM Dict28/1 -> Mux52/8
  Constant53/1 -> Mux37/1
  Constant10/1 -> Traffic Object5/1
  Constant51/1 -> Mux35/2
  Bus Selector24/6 -> Mux48/6  "<a_0 y>"
  Mux55/1 -> Mux54/9
  Bus Selector6/1 -> Mux14/1  "<t_0 x>"
  Mux7/1 -> [Traffic_Info_05]
  Traffic Object6/1 -> Terminator6/1
  Bus Selector18/1 -> Mux38/1  "<t_0 x>"
  Bus Selector3/2 -> Mux5/2  "<t_0 y>"
  Mux36/1 -> [Traffic_Info_06]
  Constant50/1 -> Mux35/1
  Constant37/1 -> Traffic Object14/1
  Constant24/1 -> Mux17/2
  Bus Selector19/1 -> Mux36/1  "<t_0 x>"
  Traffic Object1/1 -> Terminator1/1
  Constant63/1 -> Mux43/2
  Mux51/1 -> Mux50/9
  Bus Selector4/2 -> Mux7/2  "<t_0 y>"
  Bus Selector19/2 -> Mux36/2  "<t_0 y>"
  Constant21/1 -> Mux15/2
  [Traffic_Info_15] -> Mux9/16
  Traffic Object28/2 -> Bus Selector31/1
  Constant30/1 -> Traffic Object8/1
  Mux32/1 -> [Traffic_Info_18]
  Bus Selector27/2 -> Mux52/2  "<t_0 y>"
  [Traffic_Info_08] -> Mux9/9
  Bus Selector27/3 -> Mux52/3  "<v_0 x>"
  Traffic Object19/1 -> Terminator19/1
  [Traffic_Info_19] -> Mux9/20
  Bus Selector20/7 -> Mux40/7  "<r_zyx z>"
  Bus Selector18/2 -> Mux38/2  "<t_0 y>"
  Bus Selector3/1 -> Mux5/1  "<t_0 x>"
  Traffic Object12/1 -> Terminator12/1
  [Traffic_Info_01] -> Mux9/2
  Constant80/1 -> Mux53/2
  [Traffic_Info_20] -> Mux9/21
  Bus Selector11/3 -> Mux20/3  "<r_zyx z>"
  Bus Selector15/3 -> Mux28/3  "<r_zyx z>"
  Mux48/1 -> [Traffic_Info_25]
  [Traffic_Info_26] -> Mux9/27
  Bus Selector16/2 -> Mux32/2  "<t_0 y>"
  Traffic Object28/1 -> Terminator28/1
  Constant17/1 -> Mux13/1
  Constant46/1 -> Traffic Object17/1
  Bus Selector14/3 -> Mux30/3  "<r_zyx z>"
  Traffic Object19/2 -> Bus Selector19/1
  Traffic Object17/2 -> Bus Selector16/1
  Bus Selector7/2 -> Mux12/2  "<t_0 y>"
  Constant64/1 -> Traffic Object23/1
  Traffic Object17/1 -> Terminator17/1
  Bus Selector25/2 -> Mux50/2  "<t_0 y>"
  Mux37/1 -> Mux36/4
  Bus Selector10/2 -> Mux22/2  "<t_0 y>"
  Constant18/1 -> Traffic Object4/1
  Bus Selector15/1 -> Mux28/1  "<t_0 x>"
  [Traffic_Info_23] -> Mux9/24
  Constant73/1 -> Traffic Object26/1
  [Traffic_Info_09] -> Mux9/10
  [Traffic_Info_10] -> Mux9/11
  Traffic Object24/2 -> Bus Selector26/1
  Bus Selector13/3 -> Mux26/3  "<r_zyx z>"
  Bus Selector8/1 -> Mux16/1  "<t_0 x>"
  Constant52/1 -> Traffic Object19/1
  Mux2/1 -> Mux1/4

== matlab function Parking/MATLAB Function3 ==
  settings: updateMethod=DISCRETE  sampleTime=0.1
  data: traffic_info input; path_out output; success_flag output; path_len output; Ego_Global_X input; Ego_Global_Y input
function [path_out, success_flag, path_len] = rrt_star_simulink_fnc(traffic_info, Ego_Global_X, Ego_Global_Y)
%#codegen

persistent path_cached path_len_cached success_cached 
if isempty(path_cached)
    path_cached = zeros(400, 2);
    path_len_cached = 0;
    success_cached = false;
end

path_out = path_cached;
path_len = path_len_cached;
success_flag = success_cached;

if success_cached
    return;
end

MAX_NODES = 1000;
MAX_PATH_LEN = 400;
goal_radius = 8.0;
goal_sample_rate = 0.05;
eta = 3.0;

start = [Ego_Global_X, Ego_Global_Y];
goal  = [7.25, -33.2];
vehicle_size = [1.97, 4.47];
%vehicle_size = [2.1, 4.6];

map_boundary = [5.5, -4, 47.5, -3.9, 47.5, -44.9, 5.5, -44.9];
x_vals = map_boundary(1:2:end);
y_vals = map_boundary(2:2:end);
x_min = min(x_vals); x_max = max(x_vals);
y_min = min(y_vals); y_max = max(y_vals);

if mod(length(traffic_info), 5) ~= 0
    obstacles = zeros(0,5);
else
    num_obj = int32(floor(length(traffic_info)/5));
    data = reshape(traffic_info, [5, num_obj])';
    obstacles = [data(:,1), data(:,2), data(:,5), data(:,4), data(:,3)];
end

empty_node = struct('pos', zeros(1,2), 'cost', 0, 'parent', int32(0));
nodes = repmat(empty_node, MAX_NODES, 1);
nodes(1).pos = reshape(start,1,2);
node_count = int32(1);
goal_node = int32(0);

for iter = 1:500
    if rand < goal_sample_rate
        sample = goal;
    else
        sample = [x_min + rand*(x_max - x_min), y_min + rand*(y_max - y_min)];
    end

    nearest_idx = int32(1);
    min_dist = norm(nodes(1).pos - sample);
    for i = 2:node_count
        d = norm(nodes(i).pos - sample);
        if d < min_dist
            min_dist = d;
            nearest_idx = int32(i);
        end
    end

    direction = sample - nodes(nearest_idx).pos;
    dist = norm(direction);
    if dist > eta
        direction = direction / dist * eta;
    end
    new_pos = nodes(nearest_idx).pos + direction;
    new_pos = reshape(new_pos,1,2);

    if check_collision(nodes(nearest_idx).pos, new_pos, vehicle_size, obstacles)
        continue;
    end

    node_count = node_count + 1;
    if node_count > MAX_NODES
        break;
    end
    nodes(node_count).pos = new_pos;
    nodes(node_count).cost = nodes(nearest_idx).cost + dist;
    nodes(node_count).parent = nearest_idx;

    if norm(new_pos - goal) < goal_radius
        goal_node = node_count;
        break;
    end
end

if goal_node > 0
    idx = goal_node;
    i = 0;
    temp_path = zeros(MAX_PATH_LEN, 2);
    while idx > 0 && i < MAX_PATH_LEN
        i = i + 1;
        temp_path(i,:) = reshape(nodes(idx).pos,1,2);
        idx = nodes(idx).parent;
    end

    flipped = flipud(temp_path(1:i,:));

%% === Hybrid A* 전·후 직진 (동적 x-offset + y 방향 판단) ===
pre_steps  = 10;    % goal 도달 전 스텝 수
post_steps = 8;     % goal 도달 후 스텝 수
step_dist  = 0.5;   % 한 스텝 거리

% RRT* 경로의 마지막 점: goal 직전 위치
last_pos = flipped(end, :);

% 접근 방향에 따라 x-offset 결정 (좌우 판단)
if last_pos(1) < goal(1)
    % 왼쪽에서 → goal 로 접근 ⇒ 직선 구간은 goal.x - 0.5
    hybrid_x = goal(1) - 0.9;
else
    % 오른쪽에서 → goal 로 접근 ⇒ 직선 구간은 goal.x + 0.5
    hybrid_x = goal(1) + 0.9;
end

% goal 위치에 따라 y 방향 판단 (상하 방향)
if goal(2) > -36.5
    % ✅ 아래쪽에서 위로 (y 증가 방향 직선 구간)
    pre_path = [ repmat(hybrid_x, pre_steps,1), ...
                 goal(2) - step_dist*(pre_steps:-1:1)' ];

    post_path = [ repmat(hybrid_x, post_steps,1), ...
                  goal(2) + step_dist*(1:post_steps)' ];
else
    % ✅ 위쪽에서 아래로 (y 감소 방향 직선 구간)
    pre_path = [ repmat(hybrid_x, pre_steps,1), ...
                 goal(2) + step_dist*(pre_steps:-1:1)' ];

    post_path = [ repmat(hybrid_x, post_steps,1), ...
                  goal(2) - step_dist*(1:post_steps)' ];
end

% goal 지점 포함한 hybrid path 생성
hybrid_path = [pre_path; goal; post_path];

% 뒤쪽 RRT* 경로 + hybrid 직선 합치고 스무딩
raw_path    = [flipped; hybrid_path];
path_interp = smooth_path(raw_path, 0.5);

% 여기서 moving average smoothing 추가 (windowSize=5 예시)
path_interp = smooth_moving_average(path_interp, 20);
path_len    = size(path_interp,1);
path_out    = zeros(MAX_PATH_LEN, 2);
path_out(1:path_len, :) = path_interp;
success_flag = true;

% 캐싱
path_cached     = path_out;
path_len_cached = path_len;
success_cached  = true;

end
end

%% ===== 보조 함수들 =====

function collision = check_collision(p1, p2, vehicle_size, obs_list)
    collision = false;
    steps = 10;
    exception_obs = [26.5, -4, 0.1, 42.0, 0];
    for t = linspace(0,1,steps)
        pt = (1-t)*p1 + t*p2;
        yaw = atan2(p2(2)-p1(2), p2(1)-p1(1));
        veh = get_bbox(pt, yaw, vehicle_size);
        for i = 1:size(obs_list,1)
            if check_single_collision(veh, obs_list(i,:))
                collision = true; return;
            end
        end
        if check_single_collision(veh, exception_obs)
            collision = true; return;
        end
    end
end

function is_collide = check_single_collision(veh_box, obs)
    yaw_obs = obs(5);
    rear_center = obs(1:2);
    length_obs = obs(4);
    width_obs = obs(3);
    fwd_vec = [cos(yaw_obs), sin(yaw_obs)];
    center = rear_center + (length_obs/2) * fwd_vec;
    obs_box = get_bbox(center, yaw_obs, [width_obs, length_obs]);
    is_collide = box_overlap(veh_box, obs_box);
end

function box = get_bbox(center, yaw, size)
    w = size(1); h = size(2);
    dx = [ w/2, -w/2, -w/2,  w/2];
    dy = [ h/2,  h/2, -h/2, -h/2];
    R = [cos(yaw), -sin(yaw); sin(yaw), cos(yaw)];
    temp = R * [dx; dy];
    box = temp + center';
end

function overlap = box_overlap(b1, b2)
    overlap = true;
    axes = get_axes(b1, b2);
    for i = 1:size(axes,2)
        proj1 = axes(:,i)' * b1;
        proj2 = axes(:,i)' * b2;
        if max(proj1) < min(proj2) || max(proj2) < min(proj1)
            overlap = false;
            return;
        end
    end
end

function axes = get_axes(b1, b2)
    edges = [b1(:,2)-b1(:,1), b1(:,3)-b1(:,2)];
    normals = [-edges(2,:); edges(1,:)];
    axes = normals ./ vecnorm(normals);
end

function path_smooth = smooth_path(path_raw, step_size)
    if size(path_raw, 1) < 2
        path_smooth = path_raw;
        return;
    end
    dist = [0; cumsum(vecnorm(diff(path_raw), 2, 2))];
    query = 0:step_size:dist(end);
    if query(end) < dist(end)
        query(end+1) = dist(end);
    end
    x_interp = spline(dist, path_raw(:,1), query);
    y_interp = spline(dist, path_raw(:,2), query);
    path_smooth = [x_interp', y_interp'];
end

function smoothed = smooth_moving_average(path, windowSize)
    N = size(path,1);
    half = floor(windowSize/2);
    smoothed = zeros(N,2);

    for i = 1:N
        if i == 1 || i == N
            smoothed(i,:) = path(i,:);  % 시작점과 끝점은 고정
        else
            i0 = max(1, i-half);
            i1 = min(N, i+half);
            smoothed(i,:) = mean(path(i0:i1,:), 1);
        end
    end
end

== matlab function Parking/MATLAB Function4 ==
  settings: updateMethod=DISCRETE  sampleTime=0.1
  data: poly_coeff input; steering_angle output; velocity input; x_lookahead output
function [steering_angle, x_lookahead] = adaptive_pure_pursuit_from_poly_fnc(poly_coeff, velocity)
% Adaptive Pure Pursuit with dynamic lookahead based on velocity and curvature
% 입력:
%   poly_coeff : 경로 다항식 계수 [1x4] (y = ax^3 + bx^2 + cx + d)
%   velocity   : 자차 속도 [m/s]
% 출력:
%   steering_angle : 조향각 [rad]
%   x_lookahead    : lookahead 거리 [m]

    % 차량 파라미터
    L = 2.9;  % 차량 휠베이스 [m]

    % Lookahead 계산 파라미터
    Lxd = 2.5;       % 기본 lookahead [m]
    kv = 0.8;        % 속도 계수
    kc = 0.05;       % 곡률 보정 계수
    rad2deg = 180 / pi;

    % 곡률 평가 위치 (예: x=3.0)에서 곡률 추정
    x_for_curv = 3.0;
    dy_dx  = polyval(polyder(poly_coeff), x_for_curv);
    d2y_dx2 = polyval(polyder(polyder(poly_coeff)), x_for_curv);
    curvature = d2y_dx2 / (1 + dy_dx^2)^(3/2);  % 곡률

    % lookahead 거리 계산
    x_lookahead = Lxd + kv * velocity - kc * abs(curvature * rad2deg);
    x_lookahead = max(2.0, x_lookahead);  % 최소 거리 제한

    % lookahead 위치에서 목표점 좌표
    y_target = polyval(poly_coeff, x_lookahead);

    % 좌표 기반 조향각 계산 (Pure Pursuit 방식)
    alpha = atan2(y_target, x_lookahead);  % heading error
    steering_angle = atan2(2 * L * sin(alpha), x_lookahead);
end

== matlab function Parking/MATLAB Function4  ==
  settings: updateMethod=DISCRETE  sampleTime=0.1
  data: path_len input; local_waypoints_ output; goal_reached output; near_goal_zone output; waypoints input; vehicle_position input; head input; success_flag input
function [local_waypoints_, goal_reached, near_goal_zone] = global_to_local_waypoints_fnc(path_len, waypoints, vehicle_position, head, success_flag)
% 로컬 좌표계 변환 + 도착 판별 + near_goal_zone 신호 생성
% 입력:
%   path_len         : 유효한 경로 길이
%   waypoints        : 전체 경로 [400 x 2]
%   vehicle_position : [x, y]
%   head             : 자차 yaw
%   success_flag     : 경로 생성 성공 여부
% 출력:
%   local_waypoints_ : 로컬 변환 경로 [400 x 2]
%   goal_reached     : 도착 여부 (1m 이내)
%   near_goal_zone   : 남은 포인트가 4개 이하

    local_waypoints_ = zeros(500, 2);  % Simulink 고정 크기 호환
    goal_reached = false;
    near_goal_zone = false;

    if ~success_flag || path_len < 1
        return;
    end

    x_ego = vehicle_position(1);
    y_ego = vehicle_position(2);

    % --- 도착 여부 판단 (절대 거리 기준) ---
    goal_threshold = 4.5;  % [m]
    goal_point = waypoints(path_len, :);
    distance_to_goal = hypot(goal_point(1) - x_ego, goal_point(2) - y_ego);
    if distance_to_goal < goal_threshold
        goal_reached = true;
    end

    % --- 가장 가까운 waypoint 인덱스 찾기 ---
    min_dist = inf;
    closest_idx = 1;
    for i = 1:path_len
        dist = hypot(waypoints(i,1) - x_ego, waypoints(i,2) - y_ego);
        if dist < min_dist
            min_dist = dist;
            closest_idx = i;
        end
    end

    % --- near_goal_zone 판단 (남은 waypoint 개수 기준) ---
    remaining_points = path_len - closest_idx + 1;
    if remaining_points <= 30
        near_goal_zone = true;
    end

    % --- 로컬 좌표계로 변환 ---
    idx = 1;
    for i = closest_idx:path_len
        dx = waypoints(i,1) - x_ego;
        dy = waypoints(i,2) - y_ego;

        x_local = dx * cos(-head) - dy * sin(-head);
        y_local = dx * sin(-head) + dy * cos(-head);

        local_waypoints_(idx, :) = [x_local, y_local];
        idx = idx + 1;
    end
end

== matlab function Parking/MATLAB Function5 ==
  settings: updateMethod=DISCRETE  sampleTime=0.1
  data: local_waypoints input; poly_coeff output
function poly_coeff = fit_polynomial_to_waypoints_fnc(local_waypoints)
% 전방 포인트(x > 0) 중 y값 차이가 10 이하이며, y값이 -30~30 사이인 포인트만 사용

    % 1차 필터링: x > 0
    valid_idx = local_waypoints(:,1) > 0;
    filtered = local_waypoints(valid_idx, :);

    % 2차 필터링: y in [-8, 8]
    y_range_idx = abs(filtered(:,2)) <= 8;
    filtered = filtered(y_range_idx, :);

    % 앞쪽 30개만 사용
    N = min(30, size(filtered, 1));
    x = filtered(1:N, 1);
    y = filtered(1:N, 2);

    % 최소 포인트 수 확인 후 3차 다항식 피팅
    if length(x) >= 4
        poly_coeff = polyfit(x, y, 3);
    else
        poly_coeff = zeros(1, 4);
    end
end

== matlab function Parking/MATLAB Function6 ==
  settings: updateMethod=DISCRETE  sampleTime=0.1
  data: poly_coeff input; goal_reached input; near_goal_zone input; target_velocity output; success_flag input; lookahead input
function target_velocity = longitudinal_speed_control_from_poly_fnc(poly_coeff, goal_reached, near_goal_zone, success_flag, lookahead)
    V_max = 7.0;
    V_min = 2.0;
    x_for_curv = lookahead;

    % 곡률 계산
    dy_dx   = polyval(polyder(poly_coeff), x_for_curv);
    d2y_dx2 = polyval(polyder(polyder(poly_coeff)), x_for_curv);
    kappa = d2y_dx2 / (1 + dy_dx^2)^(3/2);

    % 속도 계산
    time_horizon = 3.0;
    v_from_lookahead = lookahead / time_horizon;
    v_from_curvature = V_max * exp(-5.0 * abs(kappa));
    v = min(v_from_lookahead, v_from_curvature);

    % 기본 보정
    if ~success_flag
        v = 0;
    else
        v = max(V_min, v);
    end

    if near_goal_zone
        v = min(v, 1.0);
    end

    if goal_reached
        v = 0;
    end

    % ======== 저역통과 필터 (optional) =========
    persistent prev_v
    if isempty(prev_v)
        prev_v = v;
    end

    alpha = 0.95;  % 0.85~0.95 추천 (1에 가까울수록 부드럽고 느림)
    target_velocity = alpha * prev_v + (1 - alpha) * v;
    prev_v = target_velocity;
end
